simulink model "wingLevelerSil"  (R2018a)
settings: Solver=ode45  StartTime=0.0  StopTime=inf  RelTol=1e-3
libraries: etargetslib x2, dspnetwork x2, simulink x1, sldrtlib x1
settings Model: Creator=Flight Test Lab  LastModifiedBy=alireza
settings DataIOCC: SaveFormat=StructureWithTime
settings OptimizationCC: LifeSpan=inf
settings DebuggingCC: SFExecutionAtInitializationDiag=none
settings HardwareCC: ProdBitPerSizeT=32  ProdBitPerPtrDiffT=32  ProdWordSize=32  ProdHWDeviceType=Specified
settings CodeAppCC: StateflowObjectComments=on

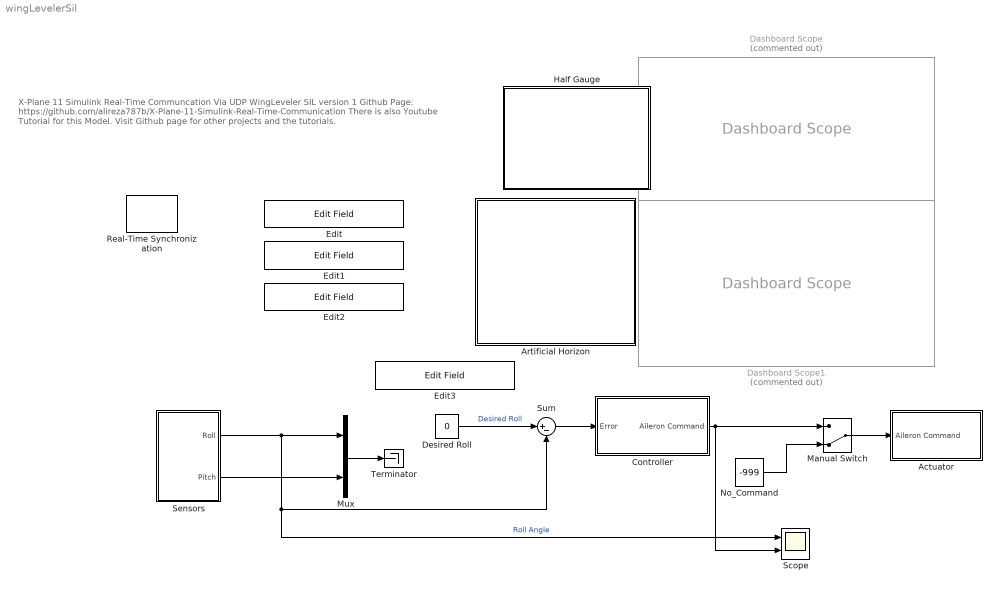
== system wingLevelerSil ==
  note: X-Plane 11 Simulink Real-Time Communcation Via UDP
      | WingLeveler SIL version 1
      | Github Page:
      | https://github.com/alireza787b/X-Plane-11-Simulink-Real-Time-Communication
      | There is also Youtube Tutorial for this Model.
      | Visit Github page for other projects and the tutorials.
  Actuator : Subsystem
  Artificial Horizon : Subsystem  DialogController=aeroblksHMICreateDDGDialog  IsWebBlock=on  mask(MWDashboardBlock){webBlockId=dbde3d10-f4c3-42da-9a7b-bdfa5df16a07, webBlockType=artificialhorizon, ShowInLibBrowser=on, ShowInitialText=on, HMISrcModelName=wingLevelerSil}
      mask prompts: webBlockId "WebBlock Id"; webBlockType "WebBlock Type"; HMISrcModelName "Source Model"
      mask help: Display aircraft attitude relative to horizon. The two signal input vector contains roll and pitch.
      mask Help: asbhmihelp('artificialhorizon')
      mask Display:
      | if strcmp(get_param(bdroot(gcb),'BlockDiagramType'), 'library')
      |  image([(matlabroot) '/toolbox/aeroblks/aeroblks/hmi/icons/ArtificialHorizonIcon.svg'])
      | end
  Controller : Subsystem
  Dashboard Scope : DashboardScope  Commented=on  ShowInitialText=off  Ymin=-100  Ymax=+100
  Dashboard Scope1 : DashboardScope  Commented=on  Ymin=-1.0  Ymax=+1.0
  Desired Roll : Constant  Value=0
  Edit : EditField  ShowInitialText=on  Alignment=Center  WebBlockId=95
  Edit1 : EditField  ShowInitialText=on  Alignment=Center  WebBlockId=96
  Edit2 : EditField  ShowInitialText=on  Alignment=Center  WebBlockId=97
  Edit3 : EditField  ShowInitialText=on  Alignment=Center  WebBlockId=103
  Half Gauge : Subsystem  DialogController=hmiCreateDDGDialog  IsWebBlock=on  mask(MWDashboardBlock){webBlockId=9dac8ba6-885d-4dd4-a2d4-b80d008318fc, webBlockType=semicirculargauge, ShowInLibBrowser=on, ShowInitialText=on, HMISrcModelName=wingLevelerSil}
      mask prompts: webBlockId "WebBlock Id"; webBlockType "WebBlock Type"; HMISrcModelName "Source Model"
      mask help: Display an input value on a semicircular scale.
      mask Help: helpview([docroot '/mapfiles/simulink.map'], 'hmi_half_gauge')
      mask Display:
      | if strcmp(get_param(bdroot(gcb),'BlockDiagramType'),'library')
      |  image([(matlabroot) '/toolbox/simulink/hmi/icons/SemiCircularGauge.png'])
      | end
  Manual Switch : ManualSwitch  CurrentSetting=0
  Mux : Mux  Inputs=2
  No_Command : Constant  Value=-999  OutDataTypeStr=single
  Real-Time Synchronization : sldrtlib/Real-Time Synchronization  SampleTime=0.05  MaxMissedTicks=10  ShowMissedTicks=off  YieldWhenWaiting=off
  Scope : Scope  NumInputPorts=2
  Sensors : Subsystem
  Sum : Sum  Inputs=|+-
  Terminator : Terminator
  wires:
  Sensors/1(Roll) -> Scope/1, Sum/2, Mux/1  "Roll Angle"
  No_Command/1 -> Manual Switch/2
  Manual Switch/1 -> Actuator/1(Aileron Command)
  Sensors/2(Pitch) -> Mux/2
  Mux/1 -> Terminator/1
  Desired Roll/1 -> Sum/1  "Desired Roll"
  Controller/1(Aileron Command) -> Manual Switch/1, Scope/2
  Sum/1 -> Controller/1(Error)

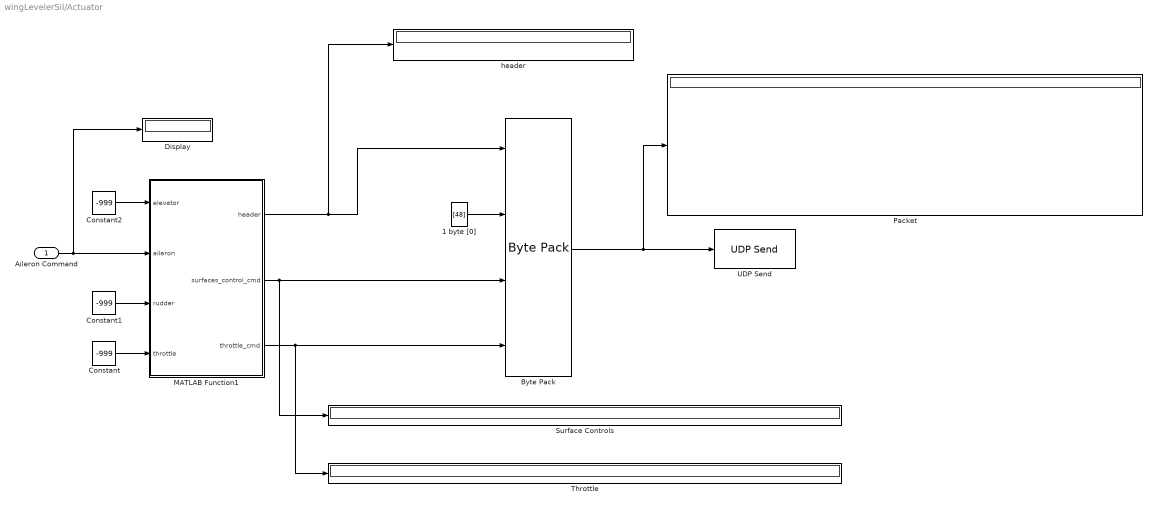
== system wingLevelerSil/Actuator ==
  Aileron Command : Inport
  1 byte [0] : Constant  Value=[48]  OutDataTypeStr=uint8
  Byte Pack : etargetslib/Byte Pack  datatypes={'uint8','uint8','single','single'}  byteAlign=1
      settings: SourceProductName=MATLAB Coder
  Constant : Constant  Value=-999  OutDataTypeStr=single
  Constant1 : Constant  Value=-999  OutDataTypeStr=single
  Constant2 : Constant  Value=-999  OutDataTypeStr=single
  Display : Display
  MATLAB Function1 : MATLAB Function  TreatAsAtomicUnit=on
  Packet : Display
  Surface Controls : Display
  Throttle : Display
  UDP Send : dspnetwork/UDP Send  remoteURL='127.0.0.1'  remotePort=49000  localURL='0.0.0.0'  localPortSource=Automatically determine  localPort=-1  sampletime=-1  blockPlatform=[]  separateLengthPort=0
      settings: SourceProductName=Simulink
  header : Display
  wires:
  MATLAB Function1/2(surfaces_control_cmd) -> Surface Controls/1, Byte Pack/3
  Byte Pack/1 -> UDP Send/1, Packet/1
  MATLAB Function1/3(throttle_cmd) -> Throttle/1, Byte Pack/4
  MATLAB Function1/1(header) -> Byte Pack/1, header/1
  Constant2/1 -> MATLAB Function1/1(elevator)
  1 byte [0]/1 -> Byte Pack/2
  Constant/1 -> MATLAB Function1/4(throttle)
  Constant1/1 -> MATLAB Function1/3(rudder)
  Aileron Command/1 -> MATLAB Function1/2(aileron), Display/1

== system wingLevelerSil/Artificial Horizon ==

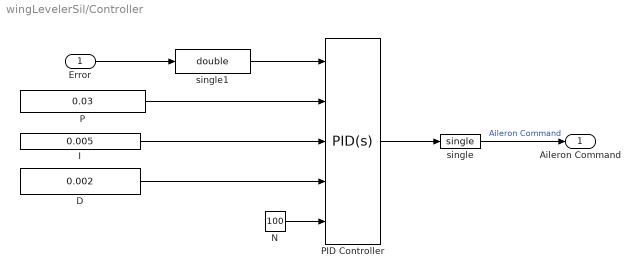
== system wingLevelerSil/Controller ==
  Error : Inport
  D : Constant  Value=0.002  OutDataTypeStr=single
  I : Constant  Value=0.005  OutDataTypeStr=single
  N : Constant  Value=100
  P : Constant  Value=0.03  OutDataTypeStr=single
  PID Controller : simulink/Continuous/PID Controller  Controller=PID  Form=Parallel  TimeDomain=Continuous-time  SampleTime=-1  IntegratorMethod=Forward Euler  FilterMethod=Forward Euler  ControllerParametersSource=external  P=-0.03  I=0  D=0  UseFilter=on  N=100  TunerSelectOption=Transfer Function Based (PID Tuner App)  InitialConditionSource=internal  InitialConditionForIntegrator=0  InitialConditionForFilter=0  DifferentiatorICPrevScaledInput=0  ExternalReset=none  TrackingMode=off  Kt=1  LimitOutput=on  UpperSaturationLimit=1  LowerSaturationLimit=-1  LinearizeAsGain=on  AntiWindupMode=back-calculation  Kb=1  POutMin=[]  POutMax=[]  IOutMin=[]  IOutMax=[]  DOutMin=[]  DOutMax=[]  NOutMin=[]  NOutMax=[]  SumOutMin=[]  SumOutMax=[]  SaturationOutMin=[]  SaturationOutMax=[]  PParamMin=[]  PParamMax=[]  IParamMin=[]  IParamMax=[]  DParamMin=[]  DParamMax=[]  NParamMin=[]  NParamMax=[]  KbParamMin=[]  KbParamMax=[]  KtParamMin=[]  KtParamMax=[]  KbOutMin=[]  KbOutMax=[]  KtOutMin=[]  KtOutMax=[]  IntegratorOutMin=[]  IntegratorOutMax=[]  FilterOutMin=[]  FilterOutMax=[]  SumI1OutMin=[]  SumI1OutMax=[]  SumI2OutMin=[]  SumI2OutMax=[]  SumI3OutMin=[]  SumI3OutMax=[]  SumDOutMin=[]  SumDOutMax=[]  DifferentiatorOutMin=[]  DifferentiatorOutMax=[]  FilterDiffOutCoefMin=[]  FilterDiffOutCoefMax=[]  ReciprocalOutMin=[]  ReciprocalOutMax=[]  SumDenOutMin=[]  SumDenOutMax=[]  SumNumOutMin=[]  SumNumOutMax=[]  DivideOutMin=[]  DivideOutMax=[]  IntegratorContinuousStateAttributes=''  IntegratorStateMustResolveToSignalObject=off  IntegratorRTWStateStorageClass=Auto  FilterContinuousStateAttributes=''  FilterStateMustResolveToSignalObject=off  FilterRTWStateStorageClass=Auto
  single : DataTypeConversion  OutDataTypeStr=single
  single1 : DataTypeConversion  OutDataTypeStr=double
  Aileron Command : Outport
  wires:
  P/1 -> PID Controller/2
  N/1 -> PID Controller/5
  I/1 -> PID Controller/3
  single/1 -> Aileron Command/1  "Aileron Command"
  PID Controller/1 -> single/1
  Error/1 -> single1/1
  D/1 -> PID Controller/4
  single1/1 -> PID Controller/1

== system wingLevelerSil/Half Gauge ==

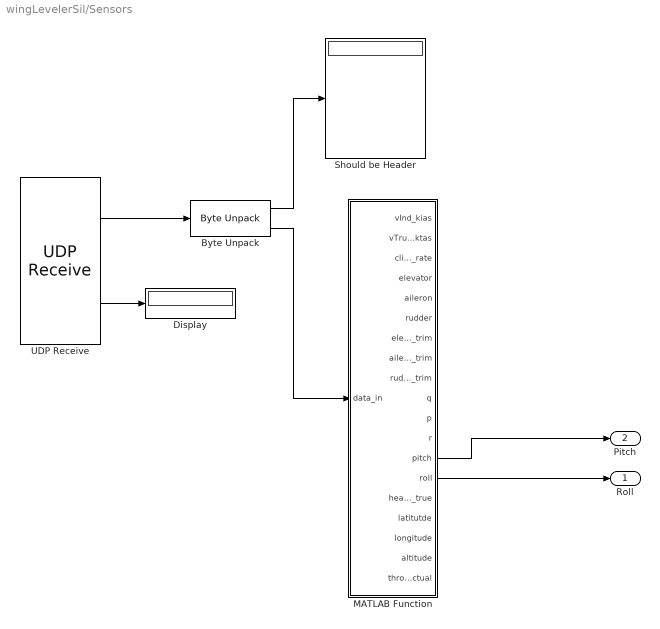
== system wingLevelerSil/Sensors ==
  Byte Unpack : etargetslib/Byte Unpack  dimensions={5,[9,8]}  datatypes={'uint8','single'}  byteAlign=1
      settings: SourceProductName=MATLAB Coder
  Display : Display
  MATLAB Function : MATLAB Function  TreatAsAtomicUnit=on
  Should be Header : Display
  UDP Receive : dspnetwork/UDP Receive  localURL='0.0.0.0'  localPort=49004  remoteURL='127.0.0.1'  remotePort=-1  recvBufferSize=8192  dims=293  signalDatatype=uint8  isVarSize=off  showBlockingTime=off  blockingTime=0  sampletime=0.05  blockPlatform=[]
      settings: SourceProductName=Simulink
  Roll : Outport
  Pitch : Outport  Port=2
  wires:
  Byte Unpack/2 -> MATLAB Function/1(data_in)
  Byte Unpack/1 -> Should be Header/1
  UDP Receive/2 -> Display/1
  UDP Receive/1 -> Byte Unpack/1
  MATLAB Function/14(roll) -> Roll/1
  MATLAB Function/13(pitch) -> Pitch/1

== matlab function wingLevelerSil/Actuator/MATLAB Function1 ==
  data: elevator input; header output uint8; surfaces_control_cmd output; aileron input single; rudder input single; throttle input; throttle_cmd output single
function [header,surfaces_control_cmd,throttle_cmd] = fcn(elevator, aileron, rudder, throttle) 
header =[uint8(68) uint8(65) uint8(84) uint8(65)];
No_Comand = single(-999);
 %Surface_header = typecast(uint8([uint8(8) uint8(0) uint8(0) uint8(0)]),'single')
surfaces_control_cmd = [1.1210388e-44 elevator aileron rudder No_Comand No_Comand No_Comand No_Comand No_Comand  ];
%Throttle_header = typecast(uint8([uint8(25) uint8(0) uint8(0) uint8(0)]),'single');
throttle_cmd = [3.503246160812043e-44 throttle No_Comand No_Comand No_Comand No_Comand No_Comand No_Comand No_Comand];
end

== matlab function wingLevelerSil/Sensors/MATLAB Function ==
  data: data_in input; vInd_kias output; vTrue_ktas output; climb_rate output; elevator output; aileron output; rudder output; elevator_trim output; aileron_trim output; rudder_trim output; q output; p output; r output; pitch output; roll output; heading_true output; latitutde output; longitude output; altitude output; throttle_actual output
function [vInd_kias,vTrue_ktas,...
    climb_rate,...
    elevator,aileron,rudder,...
    elevator_trim,aileron_trim,rudder_trim,...
    q,p,r,...
    pitch, roll, heading_true,...
    latitutde, longitude, altitude,...
    throttle_actual] = decoder(data_in)
 vInd_kias = data_in(2,1);
 vTrue_ktas = data_in(4,1);
 climb_rate = data_in(4,2);
 elevator = data_in(2,3);
 aileron = data_in(3,3);
 rudder= data_in(4,3);
 elevator_trim= data_in(2,4);
 aileron_trim= data_in(3,4);
 rudder_trim= data_in(4,4);
 q= data_in(2,5);
 p= data_in(3,5);
 r= data_in(4,5);
 pitch= data_in(2,6);
 roll= data_in(3,6);
 heading_true= data_in(4,6);
 latitutde= data_in(2,7);
 longitude= data_in(3,7);
 altitude= data_in(4,7);
 throttle_actual = data_in(2,8);
end
